simulink model "PDQuadrotor"  (R2017b)
settings: Solver=VariableStepAuto  StartTime=0.0  StopTime=10.0  RelTol=1e-3
values from neighbouring files (symbols this model uses):
  b = ()*10^(-6)    [Quadparameters.m]
  d = ()*10^(-6)    [Quadparameters.m]
  g = 9.81    [Quadparameters.m]
  Ix = 7.5*10^(-3)    (= 0.0075)    [Quadparameters.m]
  Iy = 7.5*10^(-3)    (= 0.0075)    [Quadparameters.m]
  Iz = 1.0*10^(-2)    (= 0.01)    [Quadparameters.m]
  Jr = 7.0*10^(-5)    (= 7e-05)    [Quadparameters.m]
  kdp = 0.3    [Quadparameters.m]
  kdps = 0.4    [Quadparameters.m]
  kdt = 0.3    [Quadparameters.m]
  kdz = 20    [Quadparameters.m]
  kpp = 0.7    [Quadparameters.m]
  kpps = 1    [Quadparameters.m]
  kpt = 1.1    [Quadparameters.m]
  kpz = 100    [Quadparameters.m]
  l = 0.23    [Quadparameters.m]
  m =     [Quadparameters.m]
settings Model: Creator=Jung Bae  LastModifiedBy=Jung Bae

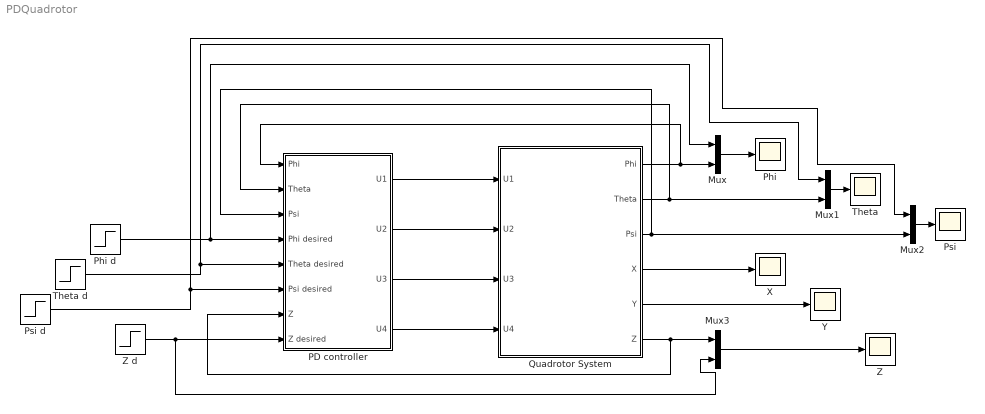
== system PDQuadrotor ==
  Mux{,1..3} (4 alike) : Mux  Inputs=2
  PD controller : Subsystem
  Phi : Scope
  Phi d : Step  SampleTime=0
  Psi : Scope
  Psi d : Step  SampleTime=0
  Quadrotor System : Subsystem
  Theta : Scope
  Theta d : Step  SampleTime=0
  X : Scope
  Y : Scope
  Z : Scope
  Z d : Step  SampleTime=0
  wires:
  Mux3/1 -> Z/1
  Z d/1 -> PD controller/8(Z desired), Mux3/2
  Quadrotor System/5(Y) -> Y/1
  Quadrotor System/1(Phi) -> PD controller/1(Phi), Mux/2
  Mux1/1 -> Theta/1
  Quadrotor System/4(X) -> X/1
  Phi d/1 -> Mux/1, PD controller/4(Phi desired)
  Mux2/1 -> Psi/1
  Psi d/1 -> PD controller/6(Psi desired), Mux2/1
  Quadrotor System/3(Psi) -> Mux2/2, PD controller/3(Psi)
  Quadrotor System/2(Theta) -> Mux1/2, PD controller/2(Theta)
  Mux/1 -> Phi/1
  Theta d/1 -> Mux1/1, PD controller/5(Theta desired)
  PD controller/3(U3) -> Quadrotor System/3(U3)
  Quadrotor System/6(Z) -> PD controller/7(Z), Mux3/1
  PD controller/4(U4) -> Quadrotor System/4(U4)
  PD controller/2(U2) -> Quadrotor System/2(U2)
  PD controller/1(U1) -> Quadrotor System/1(U1)

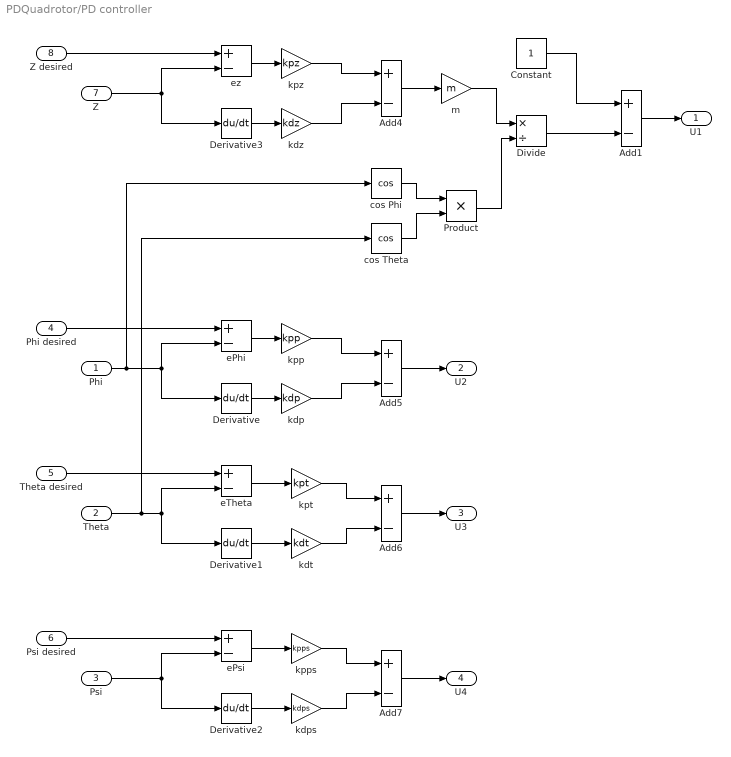
== system PDQuadrotor/PD controller ==
  Phi : Inport
  Theta : Inport  Port=2
  Psi : Inport  Port=3
  Phi desired : Inport  Port=4
  Theta desired : Inport  Port=5
  Psi desired : Inport  Port=6
  Z : Inport  Port=7
  Z desired : Inport  Port=8
  Add{1,4..7} (5 alike) : Sum  Inputs=+-
  Constant : Constant
  Derivative{,1..3} (4 alike) : Derivative
  Divide : Product  Inputs=*/
  Product : Product  RndMeth=Zero
  cos Phi : Trigonometry  Operator=cos
  cos Theta : Trigonometry  Operator=cos
  ePhi : Sum  Inputs=+-
  ePsi : Sum  Inputs=+-
  eTheta : Sum  Inputs=+-
  ez : Sum  Inputs=+-
  kdp : Gain  Gain=kdp
  kdps : Gain  Gain=kdps
  kdt : Gain  Gain=kdt
  kdz : Gain  Gain=kdz
  kpp : Gain  Gain=kpp
  kpps : Gain  Gain=kpps
  kpt : Gain  Gain=kpt
  kpz : Gain  Gain=kpz
  m : Gain  Gain=m
  U1 : Outport
  U2 : Outport  Port=2
  U3 : Outport  Port=3
  U4 : Outport  Port=4
  wires:
  Phi/1 -> Derivative/1, ePhi/2, cos Phi/1
  Theta/1 -> Derivative1/1, eTheta/2, cos Theta/1
  Psi/1 -> Derivative2/1, ePsi/2
  Phi desired/1 -> ePhi/1
  Theta desired/1 -> eTheta/1
  Psi desired/1 -> ePsi/1
  ePhi/1 -> kpp/1
  Derivative/1 -> kdp/1
  eTheta/1 -> kpt/1
  Derivative1/1 -> kdt/1
  ePsi/1 -> kpps/1
  Derivative2/1 -> kdps/1
  Z/1 -> Derivative3/1, ez/2
  Z desired/1 -> ez/1
  ez/1 -> kpz/1
  Derivative3/1 -> kdz/1
  kpz/1 -> Add4/1
  kdz/1 -> Add4/2
  kpp/1 -> Add5/1
  kdp/1 -> Add5/2
  Add5/1 -> U2/1
  kpt/1 -> Add6/1
  kdt/1 -> Add6/2
  Add6/1 -> U3/1
  kpps/1 -> Add7/1
  kdps/1 -> Add7/2
  Add7/1 -> U4/1
  cos Phi/1 -> Product/1
  cos Theta/1 -> Product/2
  Add4/1 -> m/1
  m/1 -> Divide/1
  Product/1 -> Divide/2
  Constant/1 -> Add1/1
  Divide/1 -> Add1/2
  Add1/1 -> U1/1

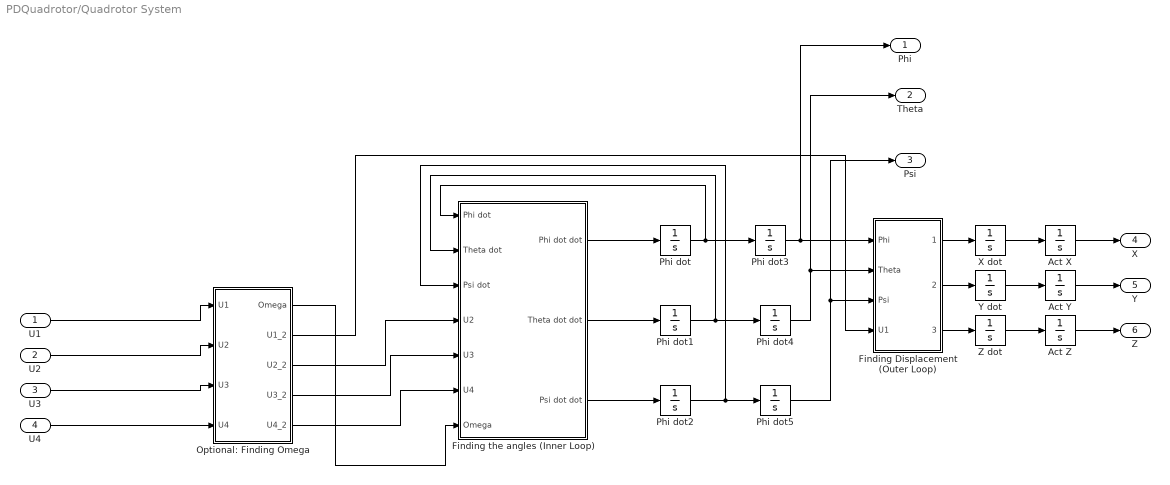
== system PDQuadrotor/Quadrotor System ==
  U1 : Inport
  U2 : Inport  Port=2
  U3 : Inport  Port=3
  U4 : Inport  Port=4
  Act X : Integrator
  Act Y : Integrator
  Act Z : Integrator
  Finding Displacement (Outer Loop) : Subsystem
  Finding the angles (Inner Loop) : Subsystem
  Optional: Finding Omega : Subsystem
  Phi dot : Integrator
  Phi dot{1..5} (5 alike) : Integrator  ZeroCross=off
  X dot : Integrator
  Y dot : Integrator
  Z dot : Integrator
  Phi : Outport
  Theta : Outport  Port=2
  Psi : Outport  Port=3
  X : Outport  Port=4
  Y : Outport  Port=5
  Z : Outport  Port=6
  wires:
  Finding the angles (Inner Loop)/1(Phi dot dot) -> Phi dot/1
  Finding the angles (Inner Loop)/2(Theta dot dot) -> Phi dot1/1
  Finding the angles (Inner Loop)/3(Psi dot dot) -> Phi dot2/1
  Phi dot/1 -> Finding the angles (Inner Loop)/1(Phi dot), Phi dot3/1
  Phi dot1/1 -> Finding the angles (Inner Loop)/2(Theta dot), Phi dot4/1
  Phi dot2/1 -> Finding the angles (Inner Loop)/3(Psi dot), Phi dot5/1
  Optional: Finding Omega/3(U2_2) -> Finding the angles (Inner Loop)/4(U2)
  Optional: Finding Omega/4(U3_2) -> Finding the angles (Inner Loop)/5(U3)
  Optional: Finding Omega/5(U4_2) -> Finding the angles (Inner Loop)/6(U4)
  Optional: Finding Omega/1(Omega) -> Finding the angles (Inner Loop)/7(Omega)
  Phi dot3/1 -> Finding Displacement (Outer Loop)/1(Phi), Phi/1
  Phi dot4/1 -> Finding Displacement (Outer Loop)/2(Theta), Theta/1
  Phi dot5/1 -> Finding Displacement (Outer Loop)/3(Psi), Psi/1
  Optional: Finding Omega/2(U1_2) -> Finding Displacement (Outer Loop)/4(U1)
  Finding Displacement (Outer Loop)/1(x dotdot) -> X dot/1
  X dot/1 -> Act X/1
  Y dot/1 -> Act Y/1
  Finding Displacement (Outer Loop)/2(y dotdot) -> Y dot/1
  Z dot/1 -> Act Z/1
  Finding Displacement (Outer Loop)/3(z dotdot) -> Z dot/1
  Act X/1 -> X/1
  Act Y/1 -> Y/1
  Act Z/1 -> Z/1
  U1/1 -> Optional: Finding Omega/1(U1)
  U2/1 -> Optional: Finding Omega/2(U2)
  U3/1 -> Optional: Finding Omega/3(U3)
  U4/1 -> Optional: Finding Omega/4(U4)

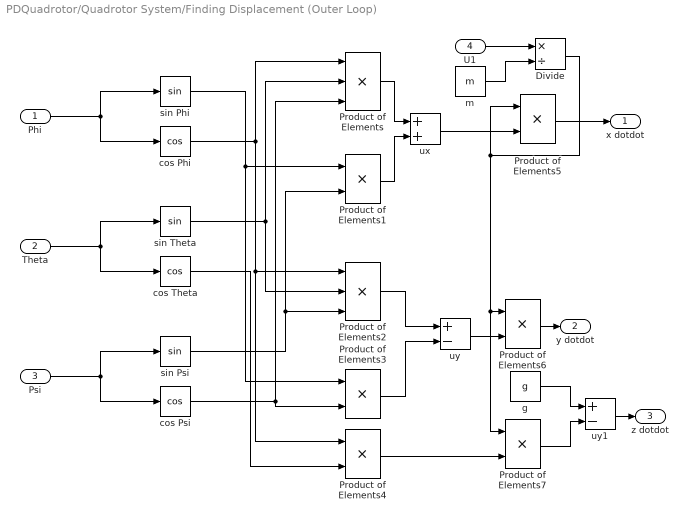
== system PDQuadrotor/Quadrotor System/Finding Displacement (Outer Loop) ==
  Phi : Inport
  Theta : Inport  Port=2
  Psi : Inport  Port=3
  U1 : Inport  Port=4
  Divide : Product  Inputs=*/
  Product of Elements : Product  Inputs=3
  Product of Elements{1,3..7} (6 alike) : Product
  Product of Elements2 : Product  Inputs=3
  cos Phi : Trigonometry  Operator=cos
  cos Psi : Trigonometry  Operator=cos
  cos Theta : Trigonometry  Operator=cos
  g : Constant  Value=g
  m : Constant  Value=m
  sin Phi : Trigonometry
  sin Psi : Trigonometry
  sin Theta : Trigonometry
  ux : Sum
  uy : Sum  Inputs=+-
  uy1 : Sum  Inputs=+-
  x dotdot : Outport
  y dotdot : Outport  Port=2
  z dotdot : Outport  Port=3
  wires:
  Phi/1 -> sin Phi/1, cos Phi/1
  Theta/1 -> sin Theta/1, cos Theta/1
  Psi/1 -> sin Psi/1, cos Psi/1
  sin Theta/1 -> Product of Elements2/2, Product of Elements/2
  cos Psi/1 -> Product of Elements3/2, Product of Elements/3
  cos Phi/1 -> Product of Elements2/1, Product of Elements4/1, Product of Elements/1
  sin Phi/1 -> Product of Elements1/1, Product of Elements3/1
  sin Psi/1 -> Product of Elements1/2, Product of Elements2/3
  Product of Elements/1 -> ux/1
  Product of Elements1/1 -> ux/2
  ux/1 -> Product of Elements5/2
  Product of Elements2/1 -> uy/1
  Product of Elements3/1 -> uy/2
  uy/1 -> Product of Elements6/2
  cos Theta/1 -> Product of Elements4/2
  Product of Elements4/1 -> Product of Elements7/2
  U1/1 -> Divide/1
  m/1 -> Divide/2
  Divide/1 -> Product of Elements5/1, Product of Elements7/1, Product of Elements6/1
  Product of Elements5/1 -> x dotdot/1
  Product of Elements6/1 -> y dotdot/1
  uy1/1 -> z dotdot/1
  Product of Elements7/1 -> uy1/2
  g/1 -> uy1/1

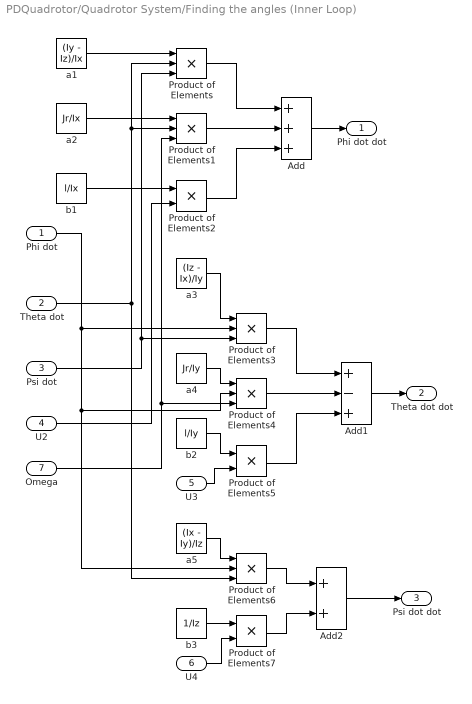
== system PDQuadrotor/Quadrotor System/Finding the angles (Inner Loop) ==
  Phi dot : Inport
  Theta dot : Inport  Port=2
  Psi dot : Inport  Port=3
  U2 : Inport  Port=4
  U3 : Inport  Port=5
  U4 : Inport  Port=6
  Omega : Inport  Port=7
  Add : Sum  Inputs=+++
  Add1 : Sum  Inputs=+-+
  Add2 : Sum
  Product of Elements{,1,3..4,6} (5 alike) : Product  Inputs=3
  Product of Elements2 : Product
  Product of Elements5 : Product
  Product of Elements7 : Product
  a1 : Constant  Value=(Iy - Iz)/Ix
  a2 : Constant  Value=Jr/Ix
  a3 : Constant  Value=(Iz - Ix)/Iy
  a4 : Constant  Value=Jr/Iy
  a5 : Constant  Value=(Ix - Iy)/Iz
  b1 : Constant  Value=l/Ix
  b2 : Constant  Value=l/Iy
  b3 : Constant  Value=1/Iz
  Phi dot dot : Outport
  Theta dot dot : Outport  Port=2
  Psi dot dot : Outport  Port=3
  wires:
  Product of Elements/1 -> Add/1
  Product of Elements1/1 -> Add/2
  Product of Elements2/1 -> Add/3
  Add/1 -> Phi dot dot/1
  a1/1 -> Product of Elements/1
  Theta dot/1 -> Product of Elements6/3, Product of Elements/2, Product of Elements1/2
  Psi dot/1 -> Product of Elements/3, Product of Elements3/3
  a2/1 -> Product of Elements1/1
  b1/1 -> Product of Elements2/1
  U2/1 -> Product of Elements2/2
  Omega/1 -> Product of Elements1/3, Product of Elements4/3
  Product of Elements3/1 -> Add1/1
  Product of Elements4/1 -> Add1/2
  Product of Elements5/1 -> Add1/3
  Add1/1 -> Theta dot dot/1
  a3/1 -> Product of Elements3/1
  a4/1 -> Product of Elements4/1
  b2/1 -> Product of Elements5/1
  U3/1 -> Product of Elements5/2
  Phi dot/1 -> Product of Elements3/2, Product of Elements4/2, Product of Elements6/2
  Product of Elements6/1 -> Add2/1
  Product of Elements7/1 -> Add2/2
  Add2/1 -> Psi dot dot/1
  U4/1 -> Product of Elements7/2
  b3/1 -> Product of Elements7/1
  a5/1 -> Product of Elements6/1

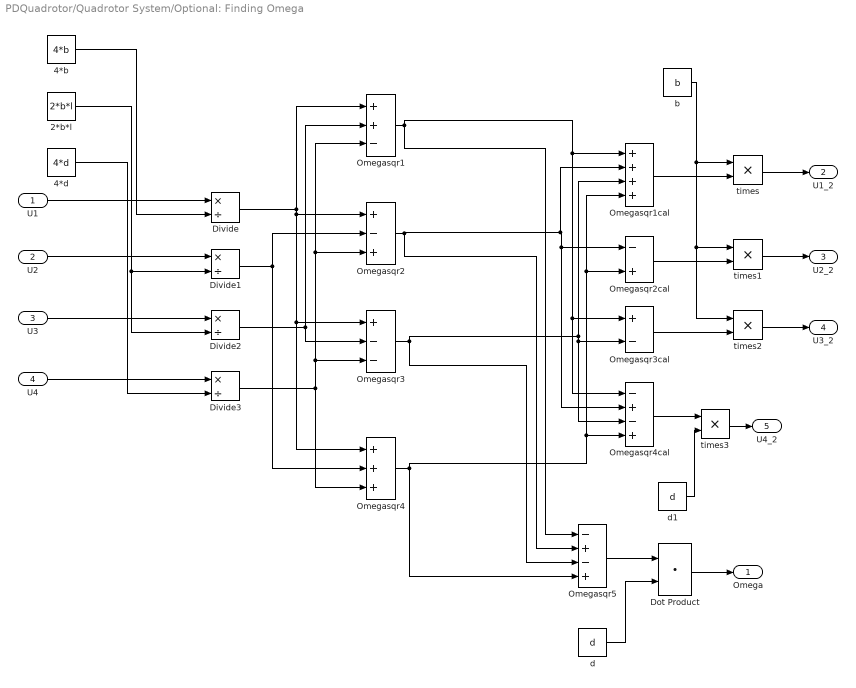
== system PDQuadrotor/Quadrotor System/Optional: Finding Omega ==
  U1 : Inport
  U2 : Inport  Port=2
  U3 : Inport  Port=3
  U4 : Inport  Port=4
  2*b*l : Constant  Value=2*b*l
  4*b : Constant  Value=4*b
  4*d : Constant  Value=4*d
  Divide{,1..3} (4 alike) : Product  Inputs=*/
  Dot Product : DotProduct  InputSameDT=on  OutDataTypeStr=Inherit: Inherit via internal rule
  Omegasqr1 : Sum  Inputs=++-
  Omegasqr1cal : Sum  Inputs=++++
  Omegasqr2 : Sum  Inputs=+-+
  Omegasqr2cal : Sum  Inputs=-+
  Omegasqr3 : Sum  Inputs=+--
  Omegasqr3cal : Sum  Inputs=+-
  Omegasqr4 : Sum  Inputs=+++
  Omegasqr4cal : Sum  Inputs=-+-+
  Omegasqr5 : Sum  Inputs=-+-+
  b : Constant  Value=b
  d : Constant  Value=d
  d1 : Constant  Value=d
  times{,1..3} (4 alike) : Product  Inputs=**
  Omega : Outport
  U1_2 : Outport  Port=2
  U2_2 : Outport  Port=3
  U3_2 : Outport  Port=4
  U4_2 : Outport  Port=5
  wires:
  U1/1 -> Divide/1
  4*b/1 -> Divide/2
  U2/1 -> Divide1/1
  2*b*l/1 -> Divide1/2, Divide2/2
  U3/1 -> Divide2/1
  U4/1 -> Divide3/1
  4*d/1 -> Divide3/2
  Divide/1 -> Omegasqr1/1, Omegasqr2/1, Omegasqr3/1, Omegasqr4/1
  Divide2/1 -> Omegasqr1/2, Omegasqr3/2
  Divide3/1 -> Omegasqr1/3, Omegasqr2/3, Omegasqr3/3, Omegasqr4/3
  Divide1/1 -> Omegasqr2/2, Omegasqr4/2
  Omegasqr1/1 -> Omegasqr4cal/1, Omegasqr3cal/1, Omegasqr1cal/1, Omegasqr5/1
  Omegasqr2/1 -> Omegasqr1cal/2, Omegasqr4cal/2, Omegasqr2cal/1, Omegasqr5/2
  Omegasqr3/1 -> Omegasqr1cal/3, Omegasqr4cal/3, Omegasqr3cal/2, Omegasqr5/3
  Omegasqr4/1 -> Omegasqr1cal/4, Omegasqr2cal/2, Omegasqr4cal/4, Omegasqr5/4
  Omegasqr5/1 -> Dot Product/1
  Dot Product/1 -> Omega/1
  d/1 -> Dot Product/2
  b/1 -> times/1, times1/1, times2/1
  Omegasqr1cal/1 -> times/2
  Omegasqr2cal/1 -> times1/2
  Omegasqr3cal/1 -> times2/2
  Omegasqr4cal/1 -> times3/1
  d1/1 -> times3/2
  times/1 -> U1_2/1
  times1/1 -> U2_2/1
  times3/1 -> U4_2/1
  times2/1 -> U3_2/1
